simulink model "batchTestIntakeIsothermal"  (R2018b)
settings: Solver=ode23t  StartTime=0.0  StopTime=3.0  MaxStep=0.1  RelTol=1e-3
libraries: nesl_utility x6, simscape_powertrain_lib x1
settings Model: SimulationMode=accelerator  Creator=264629  LastModifiedBy=grouleau
settings DataIOCC: SaveOutput=off  DSMLogging=off  SaveTime=off  SignalLoggingName=loggedSignals  OutputOption=SpecifiedOutputTimes  OutputTimes=[2 3]
settings OptimizationCC: EfficientMapNaN2IntZero=off
settings DebuggingCC: LibraryContextMissingDiagnostic=none
settings HardwareCC: TargetBitPerPointer=64  TargetBitPerSizeT=64  TargetBitPerPtrDiffT=64  TargetLongLongMode=on  TargetIntDivRoundTo=Zero  TargetEndianess=LittleEndian  TargetWordSize=64  TargetHWDeviceType=MATLAB Host  ProdEqTarget=off
settings SFSimCC: SimUseLocalCustomCode=off
settings RTWCC: RTWUseLocalCustomCode=off
settings CodeAppCC: MaxIdLength=128
settings GRTTargetCC: TargetLangStandard=C89/C90 (ANSI)  CombineOutputUpdateFcns=off  GRTInterface=on
settings SimscapeCC: SimscapeNormalizeSystem=off  SimscapeLogSimulationStatistics=on  SimscapeLogLimitData=off

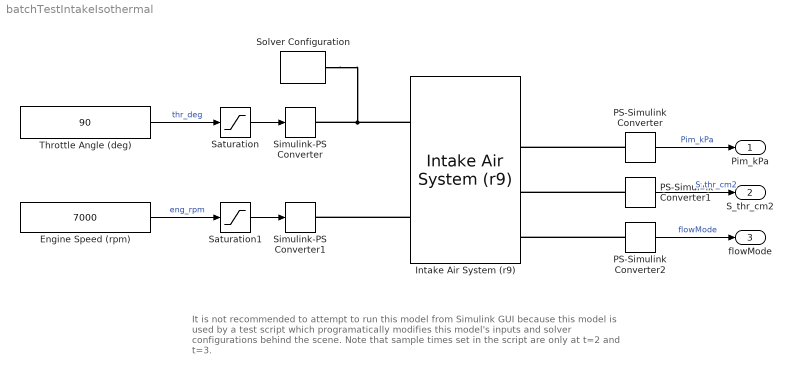
== system batchTestIntakeIsothermal ==
  note: It is not recommended to attempt to run this model from Simulink GUI
      | because this model is used by a test script which programatically modifies
      | this model's inputs and solver configurations behind the scene.
      |
      | Note that sample times set in the script are only at t=2 and t=3.
  Engine Speed (rpm) : Constant  Value=7000
  Intake Air System (r9) : simscape_powertrain_lib/engine/Intake Air System (r9)
  PS-Simulink Converter : nesl_utility/PS-Simulink Converter  PhysicalDomain=network_engine_domain  SubClassName=ps_output  LeftPortType=input  RightPortType=output  PseudoPeriodic=off  Frequencies=[]  Unit=kPa  AffineConversion=off
  PS-Simulink Converter1 : nesl_utility/PS-Simulink Converter  PhysicalDomain=network_engine_domain  SubClassName=ps_output  LeftPortType=input  RightPortType=output  PseudoPeriodic=off  Frequencies=[]  Unit=cm^2  AffineConversion=off
  PS-Simulink Converter2 : nesl_utility/PS-Simulink Converter  PhysicalDomain=network_engine_domain  SubClassName=ps_output  LeftPortType=input  RightPortType=output  PseudoPeriodic=off  Frequencies=[]  Unit=1  AffineConversion=off
  Saturation : Saturate  UpperLimit=90  LowerLimit=0
      settings: AttributesFormatString=|
      | Upper %<UpperLimit>
      | Lower %<LowerLimit>
  Saturation1 : Saturate  UpperLimit=8000  LowerLimit=0
      settings: AttributesFormatString=|
      | Upper %<UpperLimit>
      | Lower %<LowerLimit>
  Simulink-PS Converter : nesl_utility/Simulink-PS Converter  PhysicalDomain=network_engine_domain  SubClassName=ps_input  LeftPortType=input  RightPortType=output  PseudoPeriodic=off  Frequencies=[]  NoiseDistribution=none  NoiseParameters=[]  Unit=deg  AffineConversion=off  FilteringAndDerivatives=provide  SimscapeFilterOrder=1  InputFilterTimeConstant=0.001  UdotUserProvided=0
  Simulink-PS Converter1 : nesl_utility/Simulink-PS Converter  PhysicalDomain=network_engine_domain  SubClassName=ps_input  LeftPortType=input  RightPortType=output  PseudoPeriodic=off  Frequencies=[]  NoiseDistribution=none  NoiseParameters=[]  Unit=rpm  AffineConversion=off  FilteringAndDerivatives=provide  SimscapeFilterOrder=1  InputFilterTimeConstant=0.001  UdotUserProvided=0
  Solver Configuration : nesl_utility/Solver Configuration  PhysicalDomain=network_engine_domain  SubClassName=solver  LeftPortType=input  RightPortType=generic  Tones=[]  Harmonics=[]  SimulateNoise=off  Profile=off  UseLocalSampling=off  EnableSwitchedLinearOptims=on  FrequencyDomain=off  UseCCode=off  RelTol=0.001  AbsTol=1e-06  MinStep=1e-09  ToWorkspace=off  RevertToSquareIcSolve=off  NumHomotopyIterations=100  PhasorMode=off  PhasorModeNumHarmonics=1  DoDC=off  ResidualTolerance=1e-09  UseLocalSolver=off  LocalSolverChoice=NE_BACKWARD_EULER_ADVANCER  LocalSolverSampleTime=0.001  DoFixedCost=off  MaxNonlinIter=3  MaxModeIter=2  LinearAlgebra=Sparse  EquationFormulation=NE_TIME_EF  DelaysMemoryBudget=1024  AutomaticFiltering=on  FilteringTimeConstant=0.001  PartitionStorageMethod=AS_NEEDED  PartitionMemoryBudget=1024
      settings: AttributesFormatString=Local solver %<UseLocalSolver>
  Throttle Angle (deg) : Constant  Value=90
  Pim_kPa : Outport
  S_thr_cm2 : Outport  Port=2
  flowMode : Outport  Port=3
  wires:
  Throttle Angle (deg)/1 -> Saturation/1  "thr_deg"
  Engine Speed (rpm)/1 -> Saturation1/1  "eng_rpm"
  PS-Simulink Converter/1 -> Pim_kPa/1  "Pim_kPa"
  Saturation/1 -> Simulink-PS Converter/1
  Saturation1/1 -> Simulink-PS Converter1/1
  PS-Simulink Converter1/1 -> S_thr_cm2/1  "S_thr_cm2"
  PS-Simulink Converter2/1 -> flowMode/1  "flowMode"
  connections:
  Solver Configuration/RConn1 -- Intake Air System (r9)/LConn1 -- Simulink-PS Converter/RConn1
  Intake Air System (r9)/LConn2 -- Simulink-PS Converter1/RConn1
  PS-Simulink Converter2/LConn1 -- Intake Air System (r9)/RConn4
  PS-Simulink Converter1/LConn1 -- Intake Air System (r9)/RConn3
  PS-Simulink Converter/LConn1 -- Intake Air System (r9)/RConn2
